simulink model "System_Identification"  (R2022b)
settings: Solver=VariableStepAuto  StartTime=0.0  StopTime=10.0  RelTol=1e-3
values from neighbouring files (symbols this model uses):
  a = 3010.7    [DC_Motor_Parameters.m]    (also in ModellingEquation.m = X(3); Z_Domain_Parameters.m)
  b0 = -1.6285    [DC_Motor_Parameters.m]    (also in ModellingEquation.m = X(1); Z_Domain_Parameters.m)
  b1 = 0.644    [DC_Motor_Parameters.m]    (also in ModellingEquation.m = X(2); Z_Domain_Parameters.m)
  T = 4.093 * (10^(-5))    (= 4.093e-05)    [DC_Motor_Parameters.m]    (also in Z_Domain_Parameters.m)
settings Model: Creator=frz  LastModifiedBy=frz

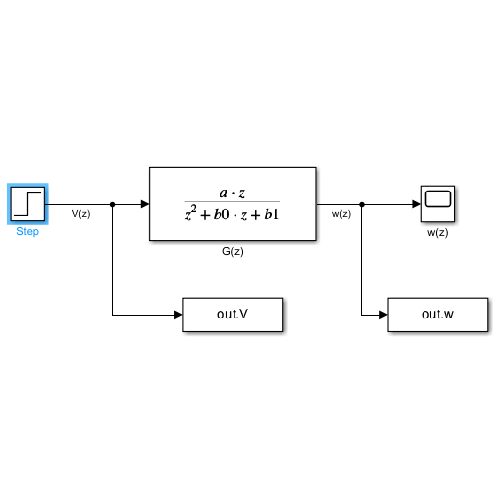
[thumbnail: Simulink's stored preview of the top-level diagram]
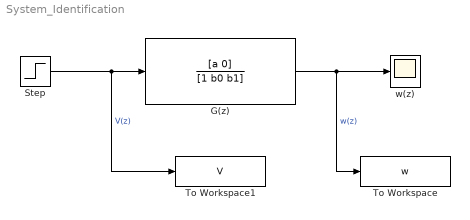
== system System_Identification ==
  G(z) : DiscreteTransferFcn  Numerator=[a 0]  Denominator=[1 b0 b1]  SampleTime=4.093e-5
  Step : Step  Time=T  After=346  SampleTime=T
  To Workspace : ToWorkspace  VariableName=w  SampleTime=T
  To Workspace1 : ToWorkspace  VariableName=V  SampleTime=T
  w(z) : Scope
  wires:
  G(z)/1 -> w(z)/1, To Workspace/1  "w(z)"
  Step/1 -> To Workspace1/1, G(z)/1  "V(z)"
